simulink model "asbQuadcopter"  (R2024b)
settings: Solver=ode3  StartTime=0  StopTime=TFinal  FixedStep=Ts  RelTol=1e-3  EnableMultiTasking=on
undefined symbols (not defined in the file): Command, Earth, ft, init, m, Rec, s, SDTV, Sim3dSensor, takeOffDuration, Ts, Vehicle, WGS84
libraries: simulink x18, sim3dlib x6, aerolibconvert2 x5, aerolibsim3d x4, aerolibanimutils x2, SignalEditorBlockLib x2, environmentLibrary x2, visionconversions x2, visiongeotforms x2, visionsinks x2, sensorsLibrary x2, aerolibfltsims x2
(part 2 of 2)

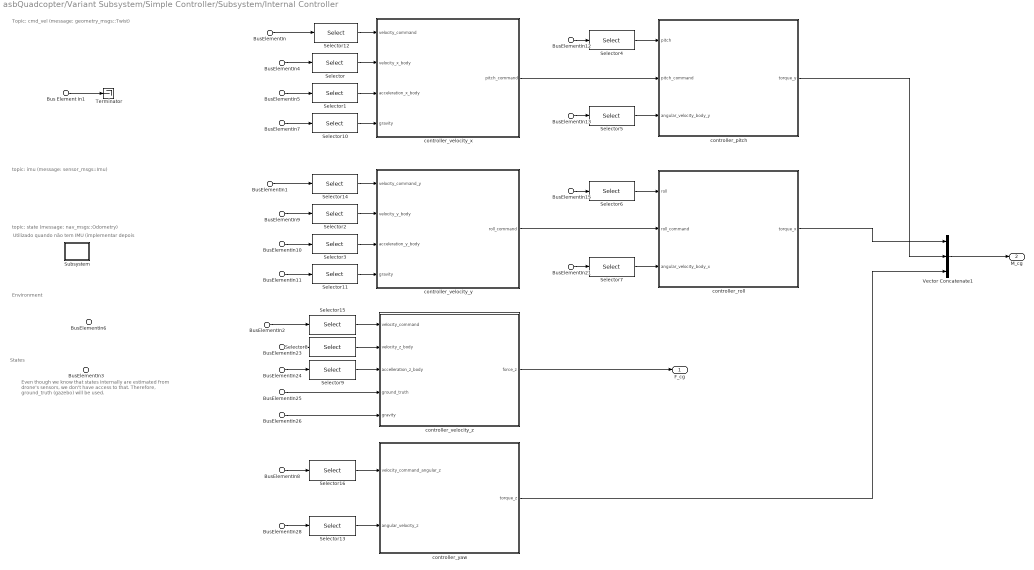
== system asbQuadcopter/Variant Subsystem/Simple Controller/Subsystem/Internal Controller ==
  note: Even though we know that states internally are estimated from drone's sensors, we don't have access to that. Therefore, ground_truth (gazebo) will be used.
  note: Utilizado quando não tem IMU (implementar depois
  note: States
  note: Topic: cmd_vel (message: geometry_msgs::Twist)
  note: topic: imu (message: sensor_msgs::Imu)
  note: topic: state (message: nav_msgs::Odometry)
  note: Environment
  Bus Element In1 : Inport  PortName=command_velocity
  BusElementIn : Inport  PortName=command_velocity  Element=linear
  BusElementIn1 : Inport  PortName=command_velocity  Element=linear
  BusElementIn2 : Inport  PortName=command_velocity  Element=linear
  BusElementIn8 : Inport  PortName=command_velocity  Element=angular
  BusElementIn6 : Inport  Port=2  PortName=environment
  BusElementIn7 : Inport  Port=2  PortName=environment  Element=Gravity_ned
  BusElementIn11 : Inport  Port=2  PortName=environment  Element=Gravity_ned
  BusElementIn26 : Inport  Port=2  PortName=environment  Element=Gravity_ned
  BusElementIn3 : Inport  Port=3  PortName=ground_truth
  BusElementIn4 : Inport  Port=3  PortName=ground_truth  Element=V_body
  BusElementIn9 : Inport  Port=3  PortName=ground_truth  Element=V_body
  BusElementIn23 : Inport  Port=3  PortName=ground_truth  Element=V_body
  BusElementIn13 : Inport  Port=3  PortName=ground_truth  Element=Omega_body
  BusElementIn28 : Inport  Port=3  PortName=ground_truth  Element=Omega_body
  BusElementIn12 : Inport  Port=3  PortName=ground_truth  Element=Euler
  BusElementIn15 : Inport  Port=3  PortName=ground_truth  Element=Euler
  BusElementIn{5,10,21,24} (4 alike) : Inport  Port=3  PortName=ground_truth  Element=Accel_body
  BusElementIn25 : Inport  Port=3  PortName=ground_truth  Element=DCM_be
  Selector{,1,6..7,12} (5 alike) : Selector  InputPortWidth=3  IndexOptions=Index vector (dialog)  Indices=1  OutputSizes=1
  Selector{8..11,13,15..16} (7 alike) : Selector  InputPortWidth=3  IndexOptions=Index vector (dialog)  Indices=3  OutputSizes=1
  Selector{2..5,14} (5 alike) : Selector  InputPortWidth=3  IndexOptions=Index vector (dialog)  Indices=2  OutputSizes=1
  Subsystem : Subsystem
  Terminator : Terminator
  Vector Concatenate1 : Concatenate  NumInputs=3
  controller_pitch : Subsystem
  controller_roll : Subsystem
  controller_velocity_x : Subsystem
  controller_velocity_y : Subsystem
  controller_velocity_z : Subsystem
  controller_yaw : Subsystem
  F_cg : Outport  Unit=N  VectorParamsAs1DForOutWhenUnconnected=off
  M_cg : Outport  Port=2  Unit=N*m  VectorParamsAs1DForOutWhenUnconnected=off
  wires:
  Vector Concatenate1/1 -> M_cg/1
  BusElementIn4/1 -> Selector/1
  Selector/1 -> controller_velocity_x/2(velocity_x_body)
  BusElementIn5/1 -> Selector1/1
  Selector1/1 -> controller_velocity_x/3(acceleration_x_body)
  BusElementIn7/1 -> Selector10/1
  BusElementIn10/1 -> Selector3/1
  BusElementIn9/1 -> Selector2/1
  Selector2/1 -> controller_velocity_y/2(velocity_y_body)
  Selector3/1 -> controller_velocity_y/3(acceleration_y_body)
  BusElementIn11/1 -> Selector11/1
  controller_velocity_x/1(pitch_command) -> controller_pitch/2(pitch_command)
  BusElementIn12/1 -> Selector4/1
  Selector4/1 -> controller_pitch/1(pitch)
  BusElementIn13/1 -> Selector5/1
  Selector5/1 -> controller_pitch/3(angular_velocity_body_y)
  Selector7/1 -> controller_roll/3(angular_velocity_body_x)
  Selector6/1 -> controller_roll/1(roll)
  controller_velocity_y/1(roll_command) -> controller_roll/2(roll_command)
  BusElementIn15/1 -> Selector6/1
  BusElementIn21/1 -> Selector7/1
  BusElementIn23/1 -> Selector8/1
  Selector8/1 -> controller_velocity_z/2(velocity_z_body)
  BusElementIn24/1 -> Selector9/1
  Selector9/1 -> controller_velocity_z/3(accelleration_z_body)
  BusElementIn25/1 -> controller_velocity_z/4(ground_truth)
  Selector10/1 -> controller_velocity_x/4(gravity)
  Selector11/1 -> controller_velocity_y/4(gravity)
  BusElementIn26/1 -> controller_velocity_z/5(gravity)
  BusElementIn28/1 -> Selector13/1
  BusElementIn8/1 -> Selector16/1
  Selector13/1 -> controller_yaw/2(angular_velocity_z)
  Bus Element In1/1 -> Terminator/1
  controller_roll/1(torque_x) -> Vector Concatenate1/1
  controller_pitch/1(torque_y) -> Vector Concatenate1/2
  controller_yaw/1(torque_z) -> Vector Concatenate1/3
  controller_velocity_z/1(force_z) -> F_cg/1
  BusElementIn/1 -> Selector12/1
  Selector12/1 -> controller_velocity_x/1(velocity_command)
  Selector14/1 -> controller_velocity_y/1(velocity_command_y)
  BusElementIn1/1 -> Selector14/1
  Selector15/1 -> controller_velocity_z/1(velocity_command)
  BusElementIn2/1 -> Selector15/1
  Selector16/1 -> controller_yaw/1(velocity_command_angular_z)

== system asbQuadcopter/Variant Subsystem/Simple Controller/Subsystem/Position on Earth ==
  Xe : Inport  Unit=m
  Flat Earth to LLA : aerolibtransform2/Flat Earth to LLA  units=Metric (MKS)  ptype=Earth (WGS84)  F=1/298.257223563  R=6378137  refPosPort=off  LL0=init.posLLA(1:2)  psi=Vehicle.PositionOnEarth.FlatEarthToLLA.xAxis
  Mux : Mux  Inputs=2
  href : Constant  Value=Vehicle.PositionOnEarth.href
  LLA : Outport  VectorParamsAs1DForOutWhenUnconnected=off
  wires:
  Mux/1 -> LLA/1
  Xe/1 -> Flat Earth to LLA/1
  Flat Earth to LLA/1 -> Mux/1
  Flat Earth to LLA/2 -> Mux/2
  href/1 -> Flat Earth to LLA/2

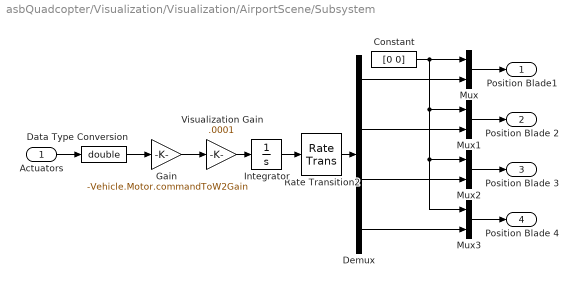
== system asbQuadcopter/Visualization/Visualization/AirportScene/Subsystem ==
  Actuators : Inport
  Constant : Constant  Value=[0 0]  VectorParams1D=off
  Data Type Conversion : DataTypeConversion  OutDataTypeStr=double  SaturateOnIntegerOverflow=off  RndMeth=Floor
  Demux : Demux
  Gain : Gain  Gain=-Vehicle.Motor.commandToW2Gain
  Integrator : Integrator  InitialCondition="[.1  .2 -.3 -.4]"  WrapState=on  WrappedStateUpperValue=2*pi  WrappedStateLowerValue=-2*pi
  Mux{,1..3} (4 alike) : Mux  Inputs=2
  Rate Transition2 : RateTransition
  Visualization Gain : Gain  Gain=.0001
  Position Blade1 : Outport  VectorParamsAs1DForOutWhenUnconnected=off
  Position Blade 2 : Outport  Port=2  VectorParamsAs1DForOutWhenUnconnected=off
  Position Blade 3 : Outport  Port=3  VectorParamsAs1DForOutWhenUnconnected=off
  Position Blade 4 : Outport  Port=4  VectorParamsAs1DForOutWhenUnconnected=off
  wires:
  Demux/4 -> Mux3/2
  Mux3/1 -> Position Blade 4/1
  Demux/2 -> Mux1/2
  Demux/3 -> Mux2/2
  Visualization Gain/1 -> Integrator/1
  Constant/1 -> Mux3/1, Mux2/1, Mux1/1, Mux/1
  Mux1/1 -> Position Blade 2/1
  Mux2/1 -> Position Blade 3/1
  Data Type Conversion/1 -> Gain/1
  Integrator/1 -> Rate Transition2/1
  Mux/1 -> Position Blade1/1
  Gain/1 -> Visualization Gain/1
  Demux/1 -> Mux/2
  Actuators/1 -> Data Type Conversion/1
  Rate Transition2/1 -> Demux/1

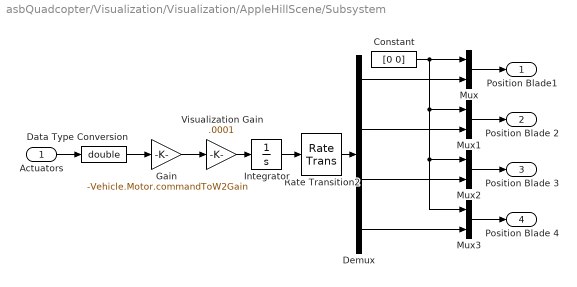
== system asbQuadcopter/Visualization/Visualization/AppleHillScene/Subsystem ==
  Actuators : Inport
  Constant : Constant  Value=[0 0]  VectorParams1D=off
  Data Type Conversion : DataTypeConversion  OutDataTypeStr=double  SaturateOnIntegerOverflow=off  RndMeth=Floor
  Demux : Demux
  Gain : Gain  Gain=-Vehicle.Motor.commandToW2Gain
  Integrator : Integrator  InitialCondition="[.1  .2 -.3 -.4]"  WrapState=on  WrappedStateUpperValue=2*pi  WrappedStateLowerValue=-2*pi
  Mux{,1..3} (4 alike) : Mux  Inputs=2
  Rate Transition2 : RateTransition
  Visualization Gain : Gain  Gain=.0001
  Position Blade1 : Outport  VectorParamsAs1DForOutWhenUnconnected=off
  Position Blade 2 : Outport  Port=2  VectorParamsAs1DForOutWhenUnconnected=off
  Position Blade 3 : Outport  Port=3  VectorParamsAs1DForOutWhenUnconnected=off
  Position Blade 4 : Outport  Port=4  VectorParamsAs1DForOutWhenUnconnected=off
  wires:
  Demux/4 -> Mux3/2
  Mux3/1 -> Position Blade 4/1
  Demux/2 -> Mux1/2
  Demux/3 -> Mux2/2
  Visualization Gain/1 -> Integrator/1
  Constant/1 -> Mux3/1, Mux2/1, Mux1/1, Mux/1
  Mux1/1 -> Position Blade 2/1
  Mux2/1 -> Position Blade 3/1
  Data Type Conversion/1 -> Gain/1
  Integrator/1 -> Rate Transition2/1
  Mux/1 -> Position Blade1/1
  Gain/1 -> Visualization Gain/1
  Demux/1 -> Mux/2
  Actuators/1 -> Data Type Conversion/1
  Rate Transition2/1 -> Demux/1

== system asbQuadcopter/Variant Subsystem/Simple Controller/Subsystem/Internal Controller/Subsystem ==
  note: void GazeboQuadrotorSimpleController::StateCallback(const nav_msgs::OdometryConstPtr& state)
      | {
      | #if (GAZEBO_MAJOR_VERSION >= 8)
      |   ignition::math::Vector3d velocity1(velocity);
      | #else
      |   math::Vector3 velocity1(velocity);
      | #endif
      |
      |   if (imu_topic_.empty()) {
      | #if (GAZEBO_MAJOR_VERSION >= 8)
      |     pose.Pos().Set(state->pose.pose.position.x, state->pose.pose.position.y, state->pose.pose.position.z);
      |     pose.Rot().Set(state->pose.pose.orientation.w, state->pose.pose.orientation.x, state->pose.pose.orientation.y, state->pose.pose.orientation.z);
      |     euler = pose.Rot().Euler();
      | #else
      |     pose.pos.Set(state->pose.pose.position.x, state->pose.pose.position.y, state->pose.pose.position.z);
      |     pose.rot.Set(state->pose.pose.orientation.w, state->pose.pose.orientation.x, state->pose.pose.orientation.y, state->pose.pose.orientation.z);
      |     euler = pose.rot.GetAsEuler();
      | #endif
      |     angular_velocity.Set(state->twist.twist.angular.x, state->twist.twist.angular.y, state->twist.twist.angular.z);
      |   }
      |
      |   velocity.Set(state->twist.twist.linear.x, state->twist.twist.linear.y, state->twist.twist.linear.z);
      |
      |   // calculate acceleration
      |   double dt = !state_stamp.isZero() ? (state->header.stamp - state_stamp).toSec() : 0.0;
      |   state_stamp = state->header.stamp;
      |   if (dt > 0.0) {
      |     acceleration = (velocity - velocity1) / dt;
      |   } else {
      |     acceleration.Set();
      |   }
      | }

== system asbQuadcopter/Variant Subsystem/Simple Controller/Subsystem/Internal Controller/controller_pitch ==
  pitch : Inport
  pitch_command : Inport  Port=2
  angular_velocity_body_y : Inport  Port=3
  Gain : Gain  Gain=Vehicle.Airframe.inertia(1)
  PID control : Subsystem
  torque_y : Outport
  wires:
  pitch_command/1 -> PID control/1(pitch_command)
  pitch/1 -> PID control/2(pitch)
  angular_velocity_body_y/1 -> PID control/3(angular_velocity_body_y)
  PID control/1(angular_acceleration) -> Gain/1
  Gain/1 -> torque_y/1

== system asbQuadcopter/Variant Subsystem/Simple Controller/Subsystem/Internal Controller/controller_roll ==
  note: void GazeboQuadrotorSimpleController::PIDController::Load(sdf::ElementPtr _sdf, const std::string& prefix)
      | {
      |   gain_p = 0.0;
      |   gain_d = 0.0;
      |   gain_i = 0.0;
      |   time_constant = 0.0;
      |   limit = -1.0;
      |
      |   if (!_sdf) return;
      |   // _sdf->PrintDescription(_sdf->GetName());
      |   if (_sdf->HasElement(prefix + "ProportionalGain")) gain_p = _sdf->GetElement(prefix + "ProportionalGain")->Get<double>();
      |   if (_sdf->HasElement(prefix + "DifferentialGain")) gain_d = _sdf->GetElement(prefix + "DifferentialGain")->Get<double>();
      |   if (_sdf->HasElement(prefix + "IntegralGain"))     gain_i = _sdf->GetElement(prefix + "IntegralGain")->Get<double>();
      |   if (_sdf->HasElement(prefix + "TimeConstant"))     time_constant = _sdf->GetElement(prefix + "TimeConstant")->Get<double>();
      |   if (_sdf->HasElement(prefix + "Limit"))            limit = _sdf->GetElement(prefix + "Limit")->Get<double>();
      | }
  roll : Inport
  roll_command : Inport  Port=2
  angular_velocity_body_x : Inport  Port=3
  Gain : Gain  Gain=Vehicle.Airframe.inertia(5)
  PID control : Subsystem
  torque_x : Outport
  wires:
  roll_command/1 -> PID control/1(roll_command)
  roll/1 -> PID control/2(roll)
  angular_velocity_body_x/1 -> PID control/3(angular_velocity_body_x)
  PID control/1(angular_acceleration) -> Gain/1
  Gain/1 -> torque_x/1

== system asbQuadcopter/Variant Subsystem/Simple Controller/Subsystem/Internal Controller/controller_velocity_x ==
  Bus Element In1 : Inport  PortName=velocity_command
  velocity_x_body : Inport  Port=2
  acceleration_x_body : Inport  Port=3
  gravity : Inport  Port=4
  Divide : Product  Inputs=*/
  PID_control : Subsystem
  pitch_command : Outport
  wires:
  velocity_x_body/1 -> PID_control/2(velocity_body)
  acceleration_x_body/1 -> PID_control/3(acceleration_body)
  PID_control/1(control_out) -> Divide/1
  Divide/1 -> pitch_command/1
  gravity/1 -> Divide/2
  Bus Element In1/1 -> PID_control/1(velocity_command)

== system asbQuadcopter/Variant Subsystem/Simple Controller/Subsystem/Internal Controller/controller_velocity_y ==
  velocity_command_y : Inport
  velocity_y_body : Inport  Port=2
  acceleration_y_body : Inport  Port=3
  gravity : Inport  Port=4
  Divide : Product  Inputs=*/
  Gain : Gain  Gain=-1
  PID_control : Subsystem
  roll_command : Outport
  wires:
  PID_control/1(control_out) -> Divide/1
  gravity/1 -> Divide/2
  velocity_command_y/1 -> PID_control/1(velocity_command)
  velocity_y_body/1 -> PID_control/2(velocity_body)
  acceleration_y_body/1 -> PID_control/3(acceleration_body)
  Divide/1 -> Gain/1
  Gain/1 -> roll_command/1

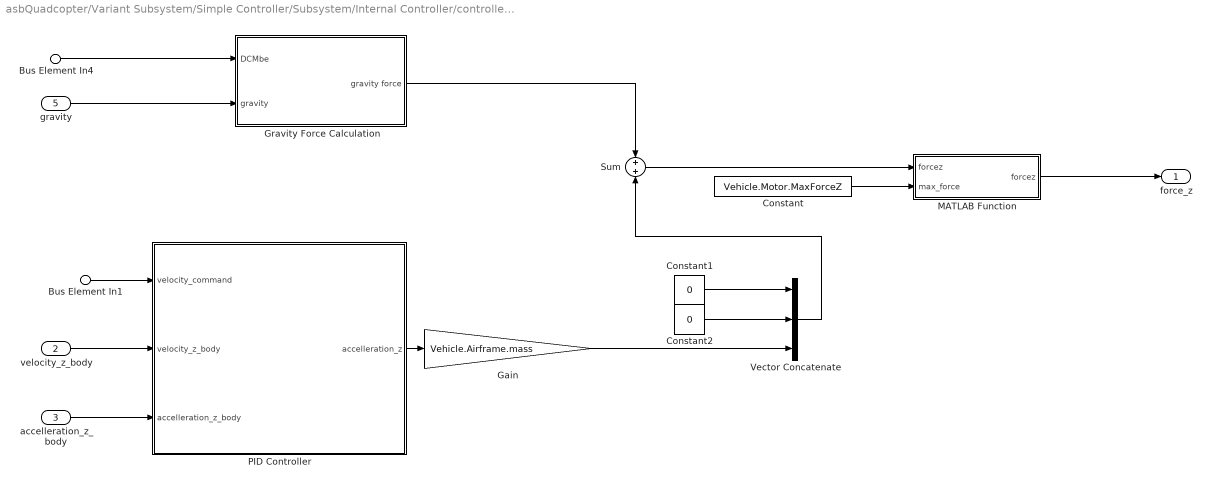
== system asbQuadcopter/Variant Subsystem/Simple Controller/Subsystem/Internal Controller/controller_velocity_z ==
  Bus Element In1 : Inport  PortName=velocity_command
  velocity_z_body : Inport  Port=2
  accelleration_z_body : Inport  Port=3
  Bus Element In4 : Inport  Port=4  PortName=ground_truth
  gravity : Inport  Port=5
  Constant : Constant  Value=Vehicle.Motor.MaxForceZ
  Constant1 : Constant  Value=0
  Constant2 : Constant  Value=0
  Gain : Gain  Gain=Vehicle.Airframe.mass
  Gravity Force Calculation : Subsystem
  MATLAB Function : MATLAB Function  TreatAsAtomicUnit=on
  PID Controller : Subsystem
  Sum : Sum
  Vector Concatenate : Concatenate  NumInputs=3
  force_z : Outport
  wires:
  MATLAB Function/1(forcez) -> force_z/1
  Bus Element In4/1 -> Gravity Force Calculation/1(DCMbe)
  gravity/1 -> Gravity Force Calculation/2(gravity)
  Bus Element In1/1 -> PID Controller/1(velocity_command)
  velocity_z_body/1 -> PID Controller/2(velocity_z_body)
  accelleration_z_body/1 -> PID Controller/3(accelleration_z_body)
  PID Controller/1(accelleration_z) -> Gain/1
  Gravity Force Calculation/1(gravity force) -> Sum/1
  Sum/1 -> MATLAB Function/1("forcez ")
  Constant/1 -> MATLAB Function/2(max_force)
  Gain/1 -> Vector Concatenate/3
  Vector Concatenate/1 -> Sum/2
  Constant1/1 -> Vector Concatenate/1
  Constant2/1 -> Vector Concatenate/2

== system asbQuadcopter/Variant Subsystem/Simple Controller/Subsystem/Internal Controller/controller_yaw ==
  velocity_command_angular_z : Inport
  angular_velocity_z : Inport  Port=2
  Constant : Constant  Value=0
  Gain : Gain  Gain=Vehicle.Airframe.inertia(9)
  PID Controller : Subsystem
  torque_z : Outport
  wires:
  velocity_command_angular_z/1 -> PID Controller/1(velocity_angular_z_command)
  angular_velocity_z/1 -> PID Controller/2(velocity_angular_z_body)
  Constant/1 -> PID Controller/3(accelleration_angular_z_body)
  PID Controller/1(accelleration_angular_z) -> Gain/1
  Gain/1 -> torque_z/1

== system asbQuadcopter/Variant Subsystem/Simple Controller/Subsystem/Internal Controller/controller_pitch/PID control ==
  pitch_command : Inport
  pitch : Inport  Port=2
  angular_velocity_body_y : Inport  Port=3
  angular_acceleration : Outport

== system asbQuadcopter/Variant Subsystem/Simple Controller/Subsystem/Internal Controller/controller_roll/PID control ==
  roll_command : Inport
  roll : Inport  Port=2
  angular_velocity_body_x : Inport  Port=3
  angular_acceleration : Outport

== system asbQuadcopter/Variant Subsystem/Simple Controller/Subsystem/Internal Controller/controller_velocity_x/PID_control ==
  velocity_command : Inport
  velocity_body : Inport  Port=2
  acceleration_body : Inport  Port=3
  control_out : Outport

== system asbQuadcopter/Variant Subsystem/Simple Controller/Subsystem/Internal Controller/controller_velocity_y/PID_control ==
  velocity_command : Inport
  velocity_body : Inport  Port=2
  acceleration_body : Inport  Port=3
  control_out : Outport

== system asbQuadcopter/Variant Subsystem/Simple Controller/Subsystem/Internal Controller/controller_velocity_z/Gravity Force Calculation ==
  DCMbe : Inport
  gravity : Inport  Port=2  Unit=m/s^2
  Gain1 : Gain  Gain=Vehicle.Airframe.mass
  Product : Product  Multiplication=Matrix(*)
  gravity force : Outport  Unit=N  VectorParamsAs1DForOutWhenUnconnected=off
  wires:
  gravity/1 -> Gain1/1
  Gain1/1 -> Product/2  "gravity force NED"
  Product/1 -> gravity force/1
  DCMbe/1 -> Product/1

== system asbQuadcopter/Variant Subsystem/Simple Controller/Subsystem/Internal Controller/controller_velocity_z/PID Controller ==
  Bus Element In1 : Inport  PortName=velocity_command
  velocity_z_body : Inport  Port=2
  accelleration_z_body : Inport  Port=3
  accelleration_z : Outport
  wires:
  ? -> accelleration_z/1

== system asbQuadcopter/Variant Subsystem/Simple Controller/Subsystem/Internal Controller/controller_yaw/PID Controller ==
  velocity_angular_z_command : Inport
  velocity_angular_z_body : Inport  Port=2
  accelleration_angular_z_body : Inport  Port=3
  accelleration_angular_z : Outport
  wires:
  ? -> accelleration_angular_z/1

== matlab function asbQuadcopter/Variant Subsystem/Simple Controller/Subsystem/Internal Controller/controller_velocity_z/MATLAB Function ==
  data: forcez input; forcez output; max_force input
function forcez = fcn(forcez,max_force)
      if (max_force > 0.0 && forcez(3) > max_force) 
          forcez(3) = max_force; 
      end
      if (forcez(3) < 0.0) 
          forcez(3) = 0.0;
      end
